simulink model "Simulazione_sistema_nl"  (R2020a)
settings: Solver=VariableStepAuto  StartTime=0.0  StopTime=(p+1)*Ts  RelTol=1e-3
values from neighbouring files (symbols this model uses):
  reg = ss(A+B*K+L*C,-L,-K,0)    [Ascensione.m]    (also in Sistema.m)
  u_max = 600    [Pianificazione_senza_vincoli.m]    (also in Pianificazione_vincoli_ingresso.m)
  u_min = -u_eq(1)    [Pianificazione_senza_vincoli.m]    (also in Pianificazione_vincoli_ingresso.m)
  x_0 = [0 0 0].'    [Pianificazione_senza_vincoli.m]
settings Model: Creator=andre  LastModifiedBy=andre
settings DataIOCC: ReturnWorkspaceOutputs=off

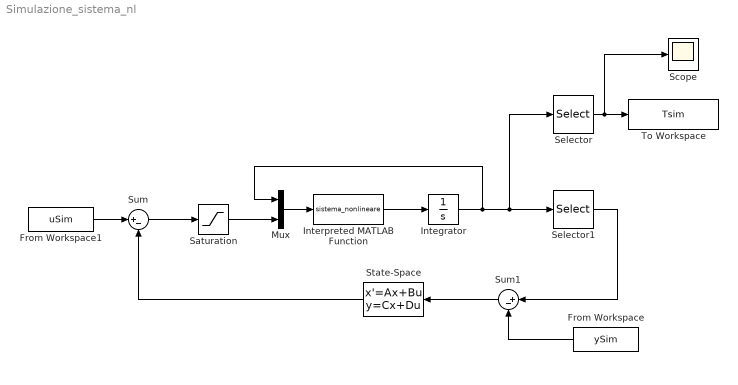
== system Simulazione_sistema_nl ==
  From Workspace : FromWorkspace  VariableName=ySim  OutputAfterFinalValue=Holding final value
  From Workspace1 : FromWorkspace  VariableName=uSim  OutputAfterFinalValue=Holding final value
  Integrator : Integrator  InitialCondition=x_0
  Interpreted MATLAB Function : MATLABFcn  MATLABFcn=sistema_nonlineare
  Mux : Mux  Inputs=2
  Saturation : Saturate  UpperLimit=u_max  LowerLimit=u_min
  Scope : Scope
  Selector : Selector  InputPortWidth=3  IndexOptions=Index vector (dialog)  Indices=[1]  OutputSizes=1
  Selector1 : Selector  InputPortWidth=3  IndexOptions=Index vector (dialog)  Indices=[2]  OutputSizes=1
  State-Space : StateSpace  A=reg.A  B=reg.B  C=reg.C  D=reg.D  InitialCondition=0
  Sum : Sum  Inputs=|+-
  Sum1 : Sum  Inputs=|+-
  To Workspace : ToWorkspace  VariableName=Tsim  SampleTime=-1
  wires:
  Interpreted MATLAB Function/1 -> Integrator/1
  Integrator/1 -> Selector/1, Selector1/1, Mux/1
  Mux/1 -> Interpreted MATLAB Function/1
  Selector/1 -> Scope/1, To Workspace/1
  From Workspace1/1 -> Sum/1
  State-Space/1 -> Sum/2
  Sum1/1 -> State-Space/1
  From Workspace/1 -> Sum1/2
  Selector1/1 -> Sum1/1
  Saturation/1 -> Mux/2
  Sum/1 -> Saturation/1
